simulink model "camber_control"  (R2025b)
settings: Solver=ode4  StartTime=0.0  StopTime=simin.Time.data(end)  FixedStep=0.01  RelTol=1e-3
model workspace (MAT data in the model file):
  simin.Car_CFL_q0.name = 'Car.CFL.q0'
  simin.Car_CFL_q0.unit = 'm'
  simin.Car_CFL_q0.nstates = 0
  simin.Car_CFL_q0.firststate = 0
  simin.Car_CFL_q0.data = [-0.000886241672561 -0.000917865429074 -0.000943370396271 -0.000939193181694 -0.000899850332644 -0.000822894508019 -0.000713430286851 -0.000581348023843 -0.000436899543274 -0.000289270334179 -0.000146343198139 -1.46837728607e-05 ... (6000 elements, 1x6000)]
  simin.Car_CFL_q2.name = 'Car.CFL.q2'
  simin.Car_CFL_q2.unit = 'm'
  simin.Car_CFL_q2.nstates = 0
  simin.Car_CFL_q2.firststate = 0
  simin.Car_CFL_q2.data = [0 1.19206197269e-05 4.64434779133e-05 5.49509059056e-05 2.16799271584e-05 -2.95135832857e-05 -7.40940522519e-05 -0.000103421145468 -0.000119076255942 -0.000124738915474 -0.000123357822304 -0.000117349867651 ... (6000 elements, 1x6000)]
  simin.Car_CFL_rx.name = 'Car.CFL.rx'
  simin.Car_CFL_rx.unit = 'rad'
  simin.Car_CFL_rx.nstates = 0
  simin.Car_CFL_rx.firststate = 0
  simin.Car_CFL_rx.data = [-0.00065072166035 -0.000697329873219 -0.000728137092665 -0.000743675802369 -0.000721060263459 -0.000660504738335 -0.000585128553212 -0.000514992512763 -0.000457198155345 -0.000411092391005 -0.000374412920792 -0.000345494656358 ... (6000 elements, 1x6000)]
  simin.Car_CFL_rx_kin.name = 'Car.CFL.rx_kin'
  simin.Car_CFL_rx_kin.unit = 'rad'
  simin.Car_CFL_rx_kin.nstates = 0
  simin.Car_CFL_rx_kin.firststate = 0
  simin.Car_CFL_rx_kin.data = [-0.000256283470662 -0.000262994930381 -0.000266255956376 -0.000264801376034 -0.000259094289504 -0.000244981871219 -0.000220309899305 -0.000186673511053 -0.000147291997564 -0.000105385945062 -6.36886106804e-05 -2.44687053055e-05 ... (6000 elements, 1x6000)]
  simin.Car_CFR_q0.name = 'Car.CFR.q0'
  simin.Car_CFR_q0.unit = 'm'
  simin.Car_CFR_q0.nstates = 0
  simin.Car_CFR_q0.firststate = 0
  simin.Car_CFR_q0.data = [-0.00088600104209 -0.000906234839931 -0.00091196334688 -0.000886910362169 -0.000833748606965 -0.000755003711674 -0.000651485286653 -0.00052521424368 -0.000380918907467 -0.000225870186114 -6.8379813456e-05 8.35821483633e-05 ... (6000 elements, 1x6000)]
  simin.Car_CFR_q2.name = 'Car.CFR.q2'
  simin.Car_CFR_q2.unit = 'm'
  simin.Car_CFR_q2.nstates = 0
  simin.Car_CFR_q2.firststate = 0
  simin.Car_CFR_q2.data = [0 1.19206197269e-05 4.64434779133e-05 5.49509059056e-05 2.16799271584e-05 -2.95135832857e-05 -7.40940522519e-05 -0.000103421145468 -0.000119076255942 -0.000124738915474 -0.000123357822304 -0.000117349867651 ... (6000 elements, 1x6000)]
  simin.Car_CFR_rx.name = 'Car.CFR.rx'
  simin.Car_CFR_rx.unit = 'rad'
  simin.Car_CFR_rx.nstates = 0
  simin.Car_CFR_rx.firststate = 0
  simin.Car_CFR_rx.data = [0.000650721834973 0.000686773331836 0.000667747866828 0.000635246396996 0.000626600987744 0.000641913560685 0.00065922603244 0.000660477147903 0.000641017919406 0.00060491275508 0.000558351166546 0.000506999145728 ... (6000 elements, 1x6000)]
  simin.Car_CFR_rx_kin.name = 'Car.CFR.rx_kin'
  simin.Car_CFR_rx_kin.unit = 'rad'
  simin.Car_CFR_rx_kin.nstates = 0
  simin.Car_CFR_rx_kin.firststate = 0
  simin.Car_CFR_rx_kin.data = [0.000256283325143 0.000263447727775 0.000270785414614 0.000265596871031 0.000246212730417 0.000216875007027 0.000181285664439 0.000141187847476 9.76538649411e-05 5.22338450537e-05 6.92095409249e-06 -3.62966420653e-05 ... (6000 elements, 1x6000)]
  simin.Car_CRL_q0.name = 'Car.CRL.q0'
  simin.Car_CRL_q0.unit = 'm'
  simin.Car_CRL_q0.nstates = 0
  simin.Car_CRL_q0.firststate = 0
  simin.Car_CRL_q0.data = [-0.000690113112796 -0.000714901543688 -0.00076236174209 -0.000825292314403 -0.000905930181034 -0.00100995623507 -0.00113963766489 -0.00129249203019 -0.00146282243077 -0.00164327386301 -0.00182610820048 -0.00200403272174 ... (6000 elements, 1x6000)]
  simin.Car_CRL_rx.name = 'Car.CRL.rx'
  simin.Car_CRL_rx.unit = 'rad'
  simin.Car_CRL_rx.nstates = 0
  simin.Car_CRL_rx.firststate = 0
  simin.Car_CRL_rx.data = [0.0257834587246 0.0257766991854 0.0257623307407 0.025743059814 0.0257183741778 0.0256865043193 0.0256465747952 0.0255992393941 0.0255462061614 0.0254897512496 0.0254323091358 0.0253761913627 ... (6000 elements, 1x6000)]
  simin.Car_CRL_rx_kin.name = 'Car.CRL.rx_kin'
  simin.Car_CRL_rx_kin.unit = 'rad'
  simin.Car_CRL_rx_kin.nstates = 0
  simin.Car_CRL_rx_kin.firststate = 0
  simin.Car_CRL_rx_kin.data = [0.0257834587246 0.0257766991854 0.0257623307407 0.025743059814 0.0257183741778 0.0256865043193 0.0256465747952 0.0255992393941 0.0255462061614 0.0254897512496 0.0254323091358 0.0253761913627 ... (6000 elements, 1x6000)]
  simin.Car_CRR_q0.name = 'Car.CRR.q0'
  simin.Car_CRR_q0.unit = 'm'
  simin.Car_CRR_q0.nstates = 0
  simin.Car_CRR_q0.firststate = 0
  simin.Car_CRR_q0.data = [-0.000689887441695 -0.000704726902768 -0.000737457768992 -0.000787679164205 -0.000858748855535 -0.000955924740992 -0.00108009413816 -0.0012272374006 -0.00139052153099 -0.0015617198078 -0.00173251959495 -0.00189547974151 ... (6000 elements, 1x6000)]
  simin.Car_CRR_rx.name = 'Car.CRR.rx'
  simin.Car_CRR_rx.unit = 'rad'
  simin.Car_CRR_rx.nstates = 0
  simin.Car_CRR_rx.firststate = 0
  simin.Car_CRR_rx.data = [-0.0257834605873 -0.0257794577628 -0.0257697012275 -0.0257545150816 -0.0257329326123 -0.0257032830268 -0.0256651025265 -0.0256195366383 -0.025568658486 -0.0255150310695 -0.0254612769932 -0.0254097674042 ... (6000 elements, 1x6000)]
  simin.Car_CRR_rx_kin.name = 'Car.CRR.rx_kin'
  simin.Car_CRR_rx_kin.unit = 'rad'
  simin.Car_CRR_rx_kin.nstates = 0
  simin.Car_CRR_rx_kin.firststate = 0
  simin.Car_CRR_rx_kin.data = [-0.0257834605873 -0.0257794577628 -0.0257697012275 -0.0257545150816 -0.0257329326123 -0.0257032830268 -0.0256651025265 -0.0256195366383 -0.025568658486 -0.0255150310695 -0.0254612769932 -0.0254097674042 ... (6000 elements, 1x6000)]
  simin.Car_CamberFL.name = 'Car.CamberFL'
  simin.Car_CamberFL.unit = 'rad'
  simin.Car_CamberFL.nstates = 0
  simin.Car_CamberFL.firststate = 0
  simin.Car_CamberFL.data = [0.00065072166035 0.000697329873219 0.000728137092665 0.000743675802369 0.000721060263459 0.000660504738335 0.000585128553212 0.000514992512763 0.000457198155345 0.000411092391005 0.000374412920792 0.000345494656358 ... (6000 elements, 1x6000)]
  simin.Car_CamberFR.name = 'Car.CamberFR'
  simin.Car_CamberFR.unit = 'rad'
  simin.Car_CamberFR.nstates = 0
  simin.Car_CamberFR.firststate = 0
  simin.Car_CamberFR.data = [0.000650721834973 0.000686773331836 0.000667747866828 0.000635246396996 0.000626600987744 0.000641913560685 0.00065922603244 0.000660477147903 0.000641017919406 0.00060491275508 0.000558351166546 0.000506999145728 ... (6000 elements, 1x6000)]
  simin.Car_CamberRL.name = 'Car.CamberRL'
  simin.Car_CamberRL.unit = 'rad'
  simin.Car_CamberRL.nstates = 0
  simin.Car_CamberRL.firststate = 0
  simin.Car_CamberRL.data = [-0.0257834587246 -0.0257766991854 -0.0257623307407 -0.025743059814 -0.0257183741778 -0.0256865043193 -0.0256465747952 -0.0255992393941 -0.0255462061614 -0.0254897512496 -0.0254323091358 -0.0253761913627 ... (6000 elements, 1x6000)]
  simin.Car_CamberRR.name = 'Car.CamberRR'
  simin.Car_CamberRR.unit = 'rad'
  simin.Car_CamberRR.nstates = 0
  simin.Car_CamberRR.firststate = 0
  simin.Car_CamberRR.data = [-0.0257834605873 -0.0257794577628 -0.0257697012275 -0.0257545150816 -0.0257329326123 -0.0257032830268 -0.0256651025265 -0.0256195366383 -0.025568658486 -0.0255150310695 -0.0254612769932 -0.0254097674042 ... (6000 elements, 1x6000)]
  simin.Car_DampFL_Frc.name = 'Car.DampFL.Frc'
  simin.Car_DampFL_Frc.unit = 'N'
  simin.Car_DampFL_Frc.nstates = 0
  simin.Car_DampFL_Frc.firststate = 0
  simin.Car_DampFL_Frc.data = [0 -9.93723297119 -4.40193367004 2.46527552605 8.21194553375 13.9642562866 18.4993839264 21.4081287384 22.7783069611 22.8000087738 21.6752319336 19.6104412079 ... (6000 elements, 1x6000)]
  simin.Car_DampFR_Frc.name = 'Car.DampFR.Frc'
  simin.Car_DampFR_Frc.unit = 'N'
  simin.Car_DampFR_Frc.nstates = 0
  simin.Car_DampFR_Frc.firststate = 0
  simin.Car_DampFR_Frc.data = [0 -5.6295466423 0.758005857468 5.51679039001 9.56676769257 13.4871988297 17.2829322815 20.6506958008 23.1178970337 24.3567123413 24.2942562103 23.0426483154 ... (6000 elements, 1x6000)]
  simin.Car_DampRL_Frc.name = 'Car.DampRL.Frc'
  simin.Car_DampRL_Frc.unit = 'N'
  simin.Car_DampRL_Frc.nstates = 0
  simin.Car_DampRL_Frc.firststate = 0
  simin.Car_DampRL_Frc.data = [0 -11.4901485443 -17.2899723053 -22.3062095642 -28.6704177856 -36.8323631287 -45.1161651611 -52.1466941833 -57.0556297302 -59.4691352844 -59.3767662048 -56.9993171692 ... (6000 elements, 1x6000)]
  simin.Car_DampRR_Frc.name = 'Car.DampRR.Frc'
  simin.Car_DampRR_Frc.unit = 'N'
  simin.Car_DampRR_Frc.nstates = 0
  simin.Car_DampRR_Frc.firststate = 0
  simin.Car_DampRR_Frc.data = [0 -7.11860799789 -12.5467271805 -18.5251407623 -25.9145946503 -34.8317947388 -43.3664627075 -50.1834983826 -54.5467147827 -56.1566467285 -55.1185531616 -51.7984848022 ... (6000 elements, 1x6000)]
  simin.Car_KinPitchCenter_L_x.name = 'Car.KinPitchCenter_L.x'
  simin.Car_KinPitchCenter_L_x.unit = 'm'
  simin.Car_KinPitchCenter_L_x.nstates = 0
  simin.Car_KinPitchCenter_L_x.firststate = 0
  simin.Car_KinPitchCenter_L_x.data = [0.504387140274 0.504145979881 0.502829492092 0.50243729353 0.503771483898 0.505480468273 0.506275355816 0.505792319775 0.504277765751 0.502096116543 0.499556958675 0.496920496225 ... (6000 elements, 1x6000)]
  simin.Car_KinPitchCenter_L_x_1.name = 'Car.KinPitchCenter_L.x_1'
  simin.Car_KinPitchCenter_L_x_1.unit = 'm'
  simin.Car_KinPitchCenter_L_x_1.nstates = 0
  simin.Car_KinPitchCenter_L_x_1.firststate = 0
  simin.Car_KinPitchCenter_L_x_1.data = [1.61338853836 1.59092903137 1.58962082863 1.58924043179 1.59058964252 1.59231734276 1.59313392639 1.59267413616 1.591183424 1.5890250206 1.58650791645 1.58389151096 ... (6000 elements, 1x6000)]
  simin.Car_KinPitchCenter_L_y_1.name = 'Car.KinPitchCenter_L.y_1'
  simin.Car_KinPitchCenter_L_y_1.unit = 'm'
  simin.Car_KinPitchCenter_L_y_1.nstates = 0
  simin.Car_KinPitchCenter_L_y_1.firststate = 0
  simin.Car_KinPitchCenter_L_y_1.data = [0.812810838223 0.812809169292 0.812811613083 0.812808275223 0.812796890736 0.812784671783 0.812776327133 0.812772095203 0.812770485878 0.812770247459 0.812770962715 0.812772035599 ... (6000 elements, 1x6000)]
  simin.Car_KinPitchCenter_L_z.name = 'Car.KinPitchCenter_L.z'
  simin.Car_KinPitchCenter_L_z.unit = 'm'
  simin.Car_KinPitchCenter_L_z.nstates = 0
  simin.Car_KinPitchCenter_L_z.firststate = 0
  simin.Car_KinPitchCenter_L_z.data = [0.203027188778 0.202923417091 0.202380791306 0.202208995819 0.202729135752 0.203393802047 0.203682735562 0.203450009227 0.202796339989 0.201870456338 0.200799122453 0.199689269066 ... (6000 elements, 1x6000)]
  simin.Car_KinPitchCenter_L_z_1.name = 'Car.KinPitchCenter_L.z_1'
  simin.Car_KinPitchCenter_L_z_1.unit = 'm'
  simin.Car_KinPitchCenter_L_z_1.nstates = 0
  simin.Car_KinPitchCenter_L_z_1.firststate = 0
  simin.Car_KinPitchCenter_L_z_1.data = [0.181995794177 0.181882992387 0.181306168437 0.181078404188 0.18152192235 0.182088240981 0.182257398963 0.181886732578 0.181082576513 0.18000048399 0.178774029016 0.177516147494 ... (6000 elements, 1x6000)]
  simin.Car_KinPitchCenter_R_x.name = 'Car.KinPitchCenter_R.x'
  simin.Car_KinPitchCenter_R_x.unit = 'm'
  simin.Car_KinPitchCenter_R_x.nstates = 0
  simin.Car_KinPitchCenter_R_x.firststate = 0
  simin.Car_KinPitchCenter_R_x.data = [0.504397392273 0.505248427391 0.507386863232 0.507622241974 0.505006432533 0.500874817371 0.496615886688 0.492787390947 0.489389508963 0.486331731081 0.483586013317 0.481158673763 ... (6000 elements, 1x6000)]
  simin.Car_KinPitchCenter_R_x_1.name = 'Car.KinPitchCenter_R.x_1'
  simin.Car_KinPitchCenter_R_x_1.unit = 'm'
  simin.Car_KinPitchCenter_R_x_1.nstates = 0
  simin.Car_KinPitchCenter_R_x_1.firststate = 0
  simin.Car_KinPitchCenter_R_x_1.data = [1.61339890957 1.59203147888 1.59417819977 1.59442532063 1.59182441235 1.58771181107 1.58347499371 1.57967054844 1.57629740238 1.57326376438 1.57054078579 1.56813430786 ... (6000 elements, 1x6000)]
  simin.Car_KinPitchCenter_R_y_1.name = 'Car.KinPitchCenter_R.y_1'
  simin.Car_KinPitchCenter_R_y_1.unit = 'm'
  simin.Car_KinPitchCenter_R_y_1.nstates = 0
  simin.Car_KinPitchCenter_R_y_1.firststate = 0
  simin.Car_KinPitchCenter_R_y_1.data = [-0.812810778618 -0.81280374527 -0.812789201736 -0.812784314156 -0.812790989876 -0.812801122665 -0.812808871269 -0.812813222408 -0.812815070152 -0.812815129757 -0.81281375885 -0.81281119585 ... (6000 elements, 1x6000)]
  simin.Car_KinPitchCenter_R_z.name = 'Car.KinPitchCenter_R.z'
  simin.Car_KinPitchCenter_R_z.unit = 'm'
  simin.Car_KinPitchCenter_R_z.nstates = 0
  simin.Car_KinPitchCenter_R_z.firststate = 0
  simin.Car_KinPitchCenter_R_z.data = [0.203031331301 0.203367009759 0.204212725163 0.204290360212 0.203219071031 0.201533898711 0.199791356921 0.198215171695 0.196806028485 0.195529073477 0.194375172257 0.193349123001 ... (6000 elements, 1x6000)]
  simin.Car_KinPitchCenter_R_z_1.name = 'Car.KinPitchCenter_R.z_1'
  simin.Car_KinPitchCenter_R_z_1.unit = 'm'
  simin.Car_KinPitchCenter_R_z_1.nstates = 0
  simin.Car_KinPitchCenter_R_z_1.firststate = 0
  simin.Car_KinPitchCenter_R_z_1.data = [0.181999951601 0.182334989309 0.183165609837 0.18320658803 0.1820730865 0.180297747254 0.178439259529 0.176727846265 0.175172701478 0.17374765873 0.172451332211 0.17129470408 ... (6000 elements, 1x6000)]
  simin.Car_KinRollCenter_F_x_1.name = 'Car.KinRollCenter_F.x_1'
  simin.Car_KinRollCenter_F_x_1.unit = 'm'
  simin.Car_KinRollCenter_F_x_1.nstates = 0
  simin.Car_KinRollCenter_F_x_1.firststate = 0
  simin.Car_KinRollCenter_F_x_1.data = [4.08391618729 4.06163883209 4.06161642075 4.06162166595 4.06163978577 4.06166744232 4.06170082092 4.06173610687 4.06177186966 4.06180620193 4.06183862686 4.0618686676 ... (6000 elements, 1x6000)]
  simin.Car_KinRollCenter_F_y.name = 'Car.KinRollCenter_F.y'
  simin.Car_KinRollCenter_F_y.unit = 'm'
  simin.Car_KinRollCenter_F_y.nstates = 0
  simin.Car_KinRollCenter_F_y.firststate = 0
  simin.Car_KinRollCenter_F_y.data = [2.19647540689e-06 0.000294854107779 0.00112901662942 0.0014056772925 0.000699118536431 -0.000498738780152 -0.00161035964265 -0.00237797247246 -0.00280151120387 -0.00295699504204 -0.0029179379344 -0.00274892663583 ... (6000 elements, 1x6000)]
  simin.Car_KinRollCenter_F_y_1.name = 'Car.KinRollCenter_F.y_1'
  simin.Car_KinRollCenter_F_y_1.unit = 'm'
  simin.Car_KinRollCenter_F_y_1.nstates = 0
  simin.Car_KinRollCenter_F_y_1.firststate = 0
  simin.Car_KinRollCenter_F_y_1.data = [2.197422873e-06 0.000292710261419 0.00111504783854 0.00137761724181 0.000672959838994 -0.000503810239024 -0.0015871420037 -0.002331224503 -0.00274047674611 -0.00289000780322 -0.00285091577098 -0.00268561020494 ... (6000 elements, 1x6000)]
  simin.Car_KinRollCenter_F_z.name = 'Car.KinRollCenter_F.z'
  simin.Car_KinRollCenter_F_z.unit = 'm'
  simin.Car_KinRollCenter_F_z.nstates = 0
  simin.Car_KinRollCenter_F_z.firststate = 0
  simin.Car_KinRollCenter_F_z.data = [0.106545142829 0.106592223048 0.106616981328 0.106594122946 0.106523387134 0.10640425235 0.106240332127 0.10604160279 0.105820596218 0.105590626597 0.105364337564 0.105152584612 ... (6000 elements, 1x6000)]
  simin.Car_KinRollCenter_F_z_1.name = 'Car.KinRollCenter_F.z_1'
  simin.Car_KinRollCenter_F_z_1.unit = 'm'
  simin.Car_KinRollCenter_F_z_1.nstates = 0
  simin.Car_KinRollCenter_F_z_1.firststate = 0
  simin.Car_KinRollCenter_F_z_1.data = [0.0853210985661 0.0853668823838 0.0853964090347 0.085396669805 0.0853713303804 0.0853234902024 0.0852591320872 0.0851852670312 0.0851074233651 0.085029900074 0.0849560722709 0.0848886221647 ... (6000 elements, 1x6000)]
  simin.Car_KinRollCenter_R_x_1.name = 'Car.KinRollCenter_R.x_1'
  simin.Car_KinRollCenter_R_x_1.unit = 'm'
  simin.Car_KinRollCenter_R_x_1.nstates = 0
  simin.Car_KinRollCenter_R_x_1.firststate = 0
  simin.Car_KinRollCenter_R_x_1.data = [1.10899782181 1.08677971363 1.086789608 1.08680522442 1.08682656288 1.08685445786 1.08688807487 1.08692574501 1.08696520329 1.08700454235 1.08704209328 1.08707654476 ... (6000 elements, 1x6000)]
  simin.Car_KinRollCenter_R_y.name = 'Car.KinRollCenter_R.y'
  simin.Car_KinRollCenter_R_y.unit = 'm'
  simin.Car_KinRollCenter_R_y.nstates = 0
  simin.Car_KinRollCenter_R_y.firststate = 0
  simin.Car_KinRollCenter_R_y.data = [-6.46729887421e-08 -3.79616576538e-05 -0.000128477113321 -0.000218971676077 -0.000285943562631 -0.000326405162923 -0.000350159883965 -0.000371785165044 -0.00040298118256 -0.000450946361525 -0.000519107619766 -0.000607466325164 ... (6000 elements, 1x6000)]
  simin.Car_KinRollCenter_R_y_1.name = 'Car.KinRollCenter_R.y_1'
  simin.Car_KinRollCenter_R_y_1.unit = 'm'
  simin.Car_KinRollCenter_R_y_1.nstates = 0
  simin.Car_KinRollCenter_R_y_1.firststate = 0
  simin.Car_KinRollCenter_R_y_1.data = [-6.4395990762e-08 -3.86120118492e-05 -0.000129369596834 -0.000219902343815 -0.00028688609018 -0.000327294197632 -0.000350904971128 -0.000372283160686 -0.000403118872782 -0.000450624676887 -0.000518255634233 -0.000606045883615 ... (6000 elements, 1x6000)]
  simin.Car_KinRollCenter_R_z.name = 'Car.KinRollCenter_R.z'
  simin.Car_KinRollCenter_R_z.unit = 'm'
  simin.Car_KinRollCenter_R_z.nstates = 0
  simin.Car_KinRollCenter_R_z.firststate = 0
  simin.Car_KinRollCenter_R_z.data = [0.0665587410331 0.0665603280067 0.0665664896369 0.0665797144175 0.0666007995605 0.0666303038597 0.0666679367423 0.0667121484876 0.066760532558 0.0668103843927 0.0668591335416 0.0669046789408 ... (6000 elements, 1x6000)]
  simin.Car_KinRollCenter_R_z_1.name = 'Car.KinRollCenter_R.z_1'
  simin.Car_KinRollCenter_R_z_1.unit = 'm'
  simin.Car_KinRollCenter_R_z_1.nstates = 0
  simin.Car_KinRollCenter_R_z_1.firststate = 0
  simin.Car_KinRollCenter_R_z_1.data = [0.0455666817725 0.0455627404153 0.0455382838845 0.0454909913242 0.045419190079 0.045320764184 0.0451966375113 0.0450519807637 0.0448944941163 0.0447327457368 0.0445747412741 0.0444271154702 ... (6000 elements, 1x6000)]
  simin.Car_Pitch.name = 'Car.Pitch'
  simin.Car_Pitch.unit = 'rad'
  simin.Car_Pitch.nstates = 0
  simin.Car_Pitch.firststate = 0
  simin.Car_Pitch.data = [-7.79904221417e-05 -7.52850028221e-05 -6.04344786552e-05 -2.87524653686e-05 2.16342832573e-05 9.28552399273e-05 0.000184569405974 0.000292906479444 0.000411794229876 0.000534347142093 0.000654049625155 0.000765463977586 ... (6000 elements, 1x6000)]
  simin.Car_PitchAcc.name = 'Car.PitchAcc'
  simin.Car_PitchAcc.unit = 'rad/s^2'
  simin.Car_PitchAcc.nstates = 0
  simin.Car_PitchAcc.firststate = 0
  simin.Car_PitchAcc.data = [-0.00852889381349 0.121664509177 0.168158859015 0.183013767004 0.209344476461 0.210217341781 0.173254683614 0.112931802869 0.0432517528534 -0.0232782959938 -0.0791946575046 -0.12137915194 ... (6000 elements, 1x6000)]
  simin.Car_PitchVel.name = 'Car.PitchVel'
  simin.Car_PitchVel.unit = 'rad/s'
  simin.Car_PitchVel.nstates = 0
  simin.Car_PitchVel.firststate = 0
  simin.Car_PitchVel.data = [-8.52889388625e-06 0.000697757815942 0.00219579669647 0.00398335745558 0.00594720616937 0.0080813486129 0.0100052338094 0.0114194946364 0.0121677154675 0.0122276162729 0.0116766653955 0.0106413085014 ... (6000 elements, 1x6000)]
  simin.Car_Roll.name = 'Car.Roll'
  simin.Car_Roll.unit = 'rad'
  simin.Car_Roll.nstates = 0
  simin.Car_Roll.firststate = 0
  simin.Car_Roll.data = [1.43921411677e-07 7.30765304979e-06 1.96193504962e-05 3.09518691211e-05 3.8966009015e-05 4.36614427599e-05 4.65610137326e-05 4.95717540616e-05 5.41080044059e-05 6.10112620052e-05 7.06324863131e-05 8.28800766612e-05 ... (6000 elements, 1x6000)]
  simin.Car_RollAcc.name = 'Car.RollAcc'
  simin.Car_RollAcc.unit = 'rad/s^2'
  simin.Car_RollAcc.nstates = 0
  simin.Car_RollAcc.firststate = 0
  simin.Car_RollAcc.data = [0.135388016701 0.0584235191345 -0.00935550685972 -0.0331188887358 -0.0355286933482 -0.020376265049 -0.000107629442937 0.0145972631872 0.0234513655305 0.0274394322187 0.0268719661981 0.0224712211639 ... (6000 elements, 1x6000)]
  simin.Car_RollVel.name = 'Car.RollVel'
  simin.Car_RollVel.unit = 'rad/s'
  simin.Car_RollVel.nstates = 0
  simin.Car_RollVel.firststate = 0
  simin.Car_RollVel.data = [0.00013538802159 0.00107662170194 0.00125746871345 0.000999151030555 0.000636012176983 0.00035703877802 0.000266080634901 0.000351245660568 0.000550257274881 0.000810600584373 0.00108493550215 0.00133225508034 ... (6000 elements, 1x6000)]
  simin.Car_SlipAngleFL.name = 'Car.SlipAngleFL'
  simin.Car_SlipAngleFL.unit = 'rad'
  simin.Car_SlipAngleFL.nstates = 0
  simin.Car_SlipAngleFL.firststate = 0
  simin.Car_SlipAngleFL.data = [0.00274525093846 0.00262049841695 0.0027533150278 0.00272545171902 0.00250543863513 0.00227329134941 0.00213159737177 0.00207538134418 0.00206845672801 0.00208716187626 0.00212029693648 0.00215951306745 ... (6000 elements, 1x6000)]
  simin.Car_SlipAngleFR.name = 'Car.SlipAngleFR'
  simin.Car_SlipAngleFR.unit = 'rad'
  simin.Car_SlipAngleFR.nstates = 0
  simin.Car_SlipAngleFR.firststate = 0
  simin.Car_SlipAngleFR.data = [-0.00274524791166 -0.00241396040656 -0.00218636821955 -0.0022307287436 -0.00249595101923 -0.00277927983552 -0.00295931030996 -0.00303354393691 -0.00303959334269 -0.00300525082275 -0.00294662476517 -0.00287613342516 ... (6000 elements, 1x6000)]
  simin.Car_SlipAngleRL.name = 'Car.SlipAngleRL'
  simin.Car_SlipAngleRL.unit = 'rad'
  simin.Car_SlipAngleRL.nstates = 0
  simin.Car_SlipAngleRL.firststate = 0
  simin.Car_SlipAngleRL.data = [0.0019979889039 0.00200495659374 0.00200151791796 0.00198903609999 0.00197318592109 0.00195616809651 0.00194171629846 0.00193085568026 0.00192299752962 0.00191747827921 0.00191350083333 0.00191024434753 ... (6000 elements, 1x6000)]
  simin.Car_SlipAngleRR.name = 'Car.SlipAngleRR'
  simin.Car_SlipAngleRR.unit = 'rad'
  simin.Car_SlipAngleRR.nstates = 0
  simin.Car_SlipAngleRR.firststate = 0
  simin.Car_SlipAngleRR.data = [-0.0019979889039 -0.00195998512208 -0.00194531306624 -0.00194091035519 -0.00193618691992 -0.00192808767315 -0.0019188785227 -0.00191189511679 -0.00191012339201 -0.00191501819063 -0.00192689360119 -0.00194531341549 ... (6000 elements, 1x6000)]
  simin.Car_SpringFL_Frc.name = 'Car.SpringFL.Frc'
  simin.Car_SpringFL_Frc.unit = 'N'
  simin.Car_SpringFL_Frc.nstates = 0
  simin.Car_SpringFL_Frc.firststate = 0
  simin.Car_SpringFL_Frc.data = [3699.37353516 3698.52294922 3697.69482422 3697.71899414 3698.77563477 3700.94433594 3704.09033203 3707.92749023 3712.15332031 3716.49487305 3720.71801758 3724.62646484 ... (6000 elements, 1x6000)]
  simin.Car_SpringFR_Frc.name = 'Car.SpringFR.Frc'
  simin.Car_SpringFR_Frc.unit = 'N'
  simin.Car_SpringFR_Frc.nstates = 0
  simin.Car_SpringFR_Frc.firststate = 0
  simin.Car_SpringFR_Frc.data = [3699.37548828 3698.82446289 3698.58496094 3699.23291016 3700.70776367 3702.93188477 3705.88891602 3709.52856445 3713.71972656 3718.25366211 3722.88623047 3727.38037109 ... (6000 elements, 1x6000)]
  simin.Car_SpringRL_Frc.name = 'Car.SpringRL.Frc'
  simin.Car_SpringRL_Frc.unit = 'N'
  simin.Car_SpringRL_Frc.nstates = 0
  simin.Car_SpringRL_Frc.firststate = 0
  simin.Car_SpringRL_Frc.data = [3300.99462891 3300.13378906 3298.30322266 3295.84838867 3292.70361328 3288.64379883 3283.55737305 3277.52734375 3270.77148438 3263.57983398 3256.26245117 3249.11352539 ... (6000 elements, 1x6000)]
  simin.Car_SpringRR_Frc.name = 'Car.SpringRR.Frc'
  simin.Car_SpringRR_Frc.unit = 'N'
  simin.Car_SpringRR_Frc.nstates = 0
  simin.Car_SpringRR_Frc.firststate = 0
  simin.Car_SpringRR_Frc.data = [3300.99658203 3300.48681641 3299.24389648 3297.30957031 3294.55981445 3290.78295898 3285.91943359 3280.11450195 3273.63354492 3266.80200195 3259.95410156 3253.39257812 ... (6000 elements, 1x6000)]
  simin.Car_StabiFL_Frc.name = 'Car.StabiFL.Frc'
  simin.Car_StabiFL_Frc.unit = 'N'
  simin.Car_StabiFL_Frc.nstates = 0
  simin.Car_StabiFL_Frc.firststate = 0
  simin.Car_StabiFL_Frc.data = [7.82602728577e-06 0.138030618429 0.413827478886 0.694055497646 0.865083992481 0.867504477501 0.764490902424 0.664155781269 0.642086148262 0.72485023737 0.906963646412 1.16916048527 ... (6000 elements, 1x6000)]
  simin.Car_StabiFR_Frc.name = 'Car.StabiFR.Frc'
  simin.Car_StabiFR_Frc.unit = 'N'
  simin.Car_StabiFR_Frc.nstates = 0
  simin.Car_StabiFR_Frc.firststate = 0
  simin.Car_StabiFR_Frc.data = [-7.82602728577e-06 -0.138030618429 -0.413827478886 -0.694055497646 -0.865083992481 -0.867504477501 -0.764490902424 -0.664155781269 -0.642086148262 -0.72485023737 -0.906963646412 -1.16916048527 ... (6000 elements, 1x6000)]
  simin.Car_StabiRL_Frc.name = 'Car.StabiRL.Frc'
  simin.Car_StabiRL_Frc.unit = 'N'
  simin.Car_StabiRL_Frc.nstates = 0
  simin.Car_StabiRL_Frc.firststate = 0
  simin.Car_StabiRL_Frc.data = [9.64909268077e-05 0.131720602512 0.35206502676 0.547254264355 0.695473074913 0.801495492458 0.885083138943 0.969595432281 1.0726429224 1.20764803886 1.38378286362 1.60394978523 ... (6000 elements, 1x6000)]
  simin.Car_StabiRR_Frc.name = 'Car.StabiRR.Frc'
  simin.Car_StabiRR_Frc.unit = 'N'
  simin.Car_StabiRR_Frc.nstates = 0
  simin.Car_StabiRR_Frc.firststate = 0
  simin.Car_StabiRR_Frc.data = [-9.64909268077e-05 -0.131720602512 -0.35206502676 -0.547254264355 -0.695473074913 -0.801495492458 -0.885083138943 -0.969595432281 -1.0726429224 -1.20764803886 -1.38378286362 -1.60394978523 ... (6000 elements, 1x6000)]
  simin.Car_SteerAngleFL.name = 'Car.SteerAngleFL'
  simin.Car_SteerAngleFL.unit = 'rad'
  simin.Car_SteerAngleFL.nstates = 0
  simin.Car_SteerAngleFL.firststate = 0
  simin.Car_SteerAngleFL.data = [-0.00274520018138 -0.00261072162539 -0.00273614027537 -0.00272827874869 -0.00252113584429 -0.00227158749476 -0.0020858021453 -0.00197293353267 -0.0019090451533 -0.00187749683391 -0.00187091040425 -0.00188293971587 ... (6000 elements, 1x6000)]
  simin.Car_SteerAngleFR.name = 'Car.SteerAngleFR'
  simin.Car_SteerAngleFR.unit = 'rad'
  simin.Car_SteerAngleFR.nstates = 0
  simin.Car_SteerAngleFR.firststate = 0
  simin.Car_SteerAngleFR.data = [0.00274519715458 0.00245770136826 0.00221033743583 0.00219813152216 0.00241411244497 0.00267922622152 0.00287288380787 0.00298104900867 0.00303049129434 0.003042408498 0.00302849058062 0.0029978682287 ... (6000 elements, 1x6000)]
  simin.Car_SteerAngleRL.name = 'Car.SteerAngleRL'
  simin.Car_SteerAngleRL.unit = 'rad'
  simin.Car_SteerAngleRL.nstates = 0
  simin.Car_SteerAngleRL.firststate = 0
  simin.Car_SteerAngleRL.data = [-0.00200000009499 -0.00200000009499 -0.00200000009499 -0.00200000009499 -0.00200000009499 -0.00200000009499 -0.00200000009499 -0.00200000009499 -0.00200000009499 -0.00200000009499 -0.00200000009499 -0.00200000009499 ... (6000 elements, 1x6000)]
  simin.Car_SteerAngleRR.name = 'Car.SteerAngleRR'
  simin.Car_SteerAngleRR.unit = 'rad'
  simin.Car_SteerAngleRR.nstates = 0
  simin.Car_SteerAngleRR.firststate = 0
  simin.Car_SteerAngleRR.data = [0.00200000009499 0.00200000009499 0.00200000009499 0.00200000009499 0.00200000009499 0.00200000009499 0.00200000009499 0.00200000009499 0.00200000009499 0.00200000009499 0.00200000009499 0.00200000009499 ... (6000 elements, 1x6000)]
  simin.Car_ax.name = 'Car.ax'
  simin.Car_ax.unit = 'm/s^2'
  simin.Car_ax.nstates = 0
  simin.Car_ax.firststate = 0
  simin.Car_ax.data = [-0.457714706659 -0.534652173519 -0.662542879581 -0.741676449776 -0.843408048153 -0.914272546768 -0.900144159794 -0.82865524292 -0.726453304291 -0.619308292866 -0.523603081703 -0.446811616421 ... (6000 elements, 1x6000)]
  simin.Car_ay.name = 'Car.ay'
  simin.Car_ay.unit = 'm/s^2'
  simin.Car_ay.nstates = 0
  simin.Car_ay.firststate = 0
  simin.Car_ay.data = [0.0283882785589 -0.0120470412076 -0.0242476686835 -0.0307025741786 -0.0163070317358 0.0105119002983 0.0332782119513 0.0458651073277 0.0503795333207 0.0500719510019 0.0471589565277 0.0429927967489 ... (6000 elements, 1x6000)]
  simin.Car_az.name = 'Car.az'
  simin.Car_az.unit = 'm/s^2'
  simin.Car_az.nstates = 0
  simin.Car_az.firststate = 0
  simin.Car_az.data = [1.57921946049 0.0678593143821 0.0510049164295 0.0390680357814 0.0383200794458 0.0183836277574 0.000795689527877 -0.0124301603064 -0.020629376173 -0.0241743065417 -0.0244926121086 -0.0227019377053 ... (6000 elements, 1x6000)]
  simin.Car_tx.name = 'Car.tx'
  simin.Car_tx.unit = 'm'
  simin.Car_tx.nstates = 0
  simin.Car_tx.firststate = 0
  simin.Car_tx.data = [2.61795282364 2.84016108513 3.0623190403 3.28441166878 3.50642991066 3.72836446762 3.9502081871 4.1719622612 4.39363288879 4.61523103714 4.83676624298 5.05824899673 ... (6000 elements, 1x6000)]
  simin.Car_ty.name = 'Car.ty'
  simin.Car_ty.unit = 'm'
  simin.Car_ty.nstates = 0
  simin.Car_ty.firststate = 0
  simin.Car_ty.data = [-5.5 -5.50000047684 -5.50000143051 -5.50000524521 -5.50001192093 -5.50001955032 -5.50002574921 -5.50002813339 -5.50002622604 -5.50001955032 -5.50000762939 -5.49999141693 ... (6000 elements, 1x6000)]
  simin.Car_tz.name = 'Car.tz'
  simin.Car_tz.unit = 'm'
  simin.Car_tz.nstates = 0
  simin.Car_tz.firststate = 0
  simin.Car_tz.data = [0.625109732151 0.62511330843 0.625121891499 0.625134706497 0.625151395798 0.62517118454 0.625193357468 0.625216901302 0.625240981579 0.625264883041 0.625288069248 0.625310182571 ... (6000 elements, 1x6000)]
  simin.Car_v.name = 'Car.v'
  simin.Car_v.unit = 'm/s'
  simin.Car_v.nstates = 0
  simin.Car_v.firststate = 0
  simin.Car_v.data = [22.2222213745 22.2189311981 22.2130565643 22.2060241699 22.1982498169 22.1894168854 22.1802577972 22.1715068817 22.1636238098 22.1568069458 22.1510219574 22.1461219788 ... (6000 elements, 1x6000)]
  simin.Steer_L_q.name = 'Steer.L.q'
  simin.Steer_L_q.unit = 'm'
  simin.Steer_L_q.nstates = 0
  simin.Steer_L_q.firststate = 0
  simin.Steer_L_q.data = [0 1.19206197269e-05 4.64434779133e-05 5.49509059056e-05 2.16799271584e-05 -2.95135832857e-05 -7.40940522519e-05 -0.000103421145468 -0.000119076255942 -0.000124738915474 -0.000123357822304 -0.000117349867651 ... (6000 elements, 1x6000)]
  simin.Steer_R_q.name = 'Steer.R.q'
  simin.Steer_R_q.unit = 'm'
  simin.Steer_R_q.nstates = 0
  simin.Steer_R_q.firststate = 0
  simin.Steer_R_q.data = [0 1.19206197269e-05 4.64434779133e-05 5.49509059056e-05 2.16799271584e-05 -2.95135832857e-05 -7.40940522519e-05 -0.000103421145468 -0.000119076255942 -0.000124738915474 -0.000123357822304 -0.000117349867651 ... (6000 elements, 1x6000)]
  simin.Steer_RL_q.name = 'Steer.RL.q'
  simin.Steer_RL_q.unit = 'm'
  simin.Steer_RL_q.nstates = 0
  simin.Steer_RL_q.firststate = 0
  simin.Steer_RL_q.data = [0 0 0 0 0 0 0 0 0 0 0 0 ... (6000 elements, 1x6000)]
  simin.Steer_RR_q.name = 'Steer.RR.q'
  simin.Steer_RR_q.unit = 'm'
  simin.Steer_RR_q.nstates = 0
  simin.Steer_RR_q.firststate = 0
  simin.Steer_RR_q.data = [0 0 0 0 0 0 0 0 0 0 0 0 ... (6000 elements, 1x6000)]
  simin.Time.name = 'Time'
  simin.Time.unit = 's'
  simin.Time.nstates = 0
  simin.Time.firststate = 0
  simin.Time.data = [0 0.01 0.02 0.03 0.04 0.05 0.06 0.07 0.08 0.09 0.1 0.11 ... (6000 elements, 1x6000)]
undefined symbols (not defined in the file): camberMapFL, compression, compression_FL, compression_FR, distance_to_pitch_center_front, steer, steering_rack_displacement_FL, steering_rack_displacement_FR, track_width_front, track_width_rear, wheelbase
settings Model: DataDictionary=vehicleData.sldd  EnableAccessToBaseWorkspace=off  Creator=marce  LastModifiedBy=marcelkaminski

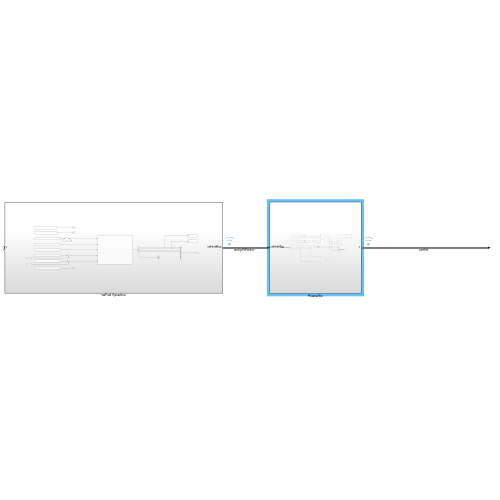
[thumbnail: Simulink's stored preview of the top-level diagram]
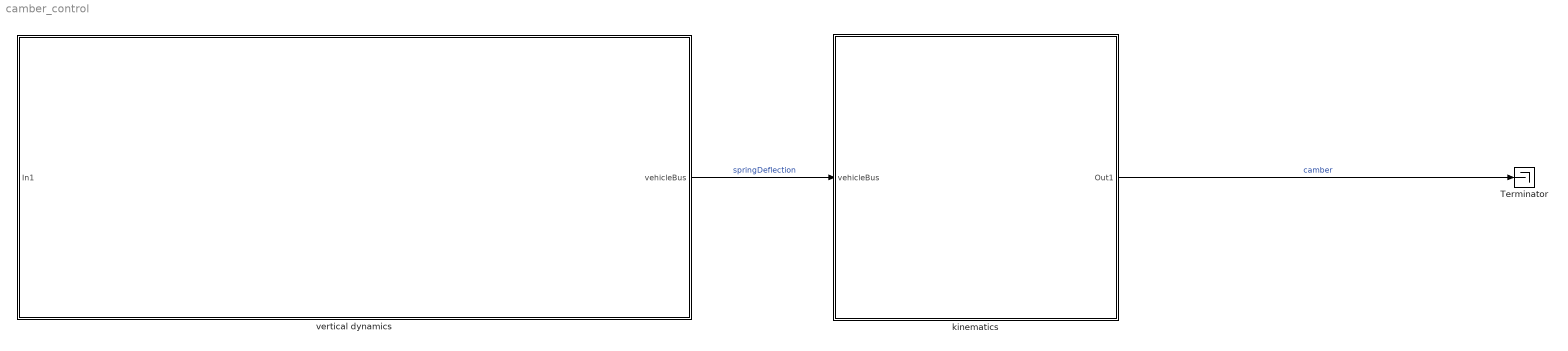
== system camber_control ==
  Terminator : Terminator
  kinematics : Subsystem
  vertical dynamics : Subsystem
  wires:
  vertical dynamics/1(vehicleBus) -> kinematics/1(vehicleBus)  "springDeflection"
  kinematics/1(Out1) -> Terminator/1  "camber"

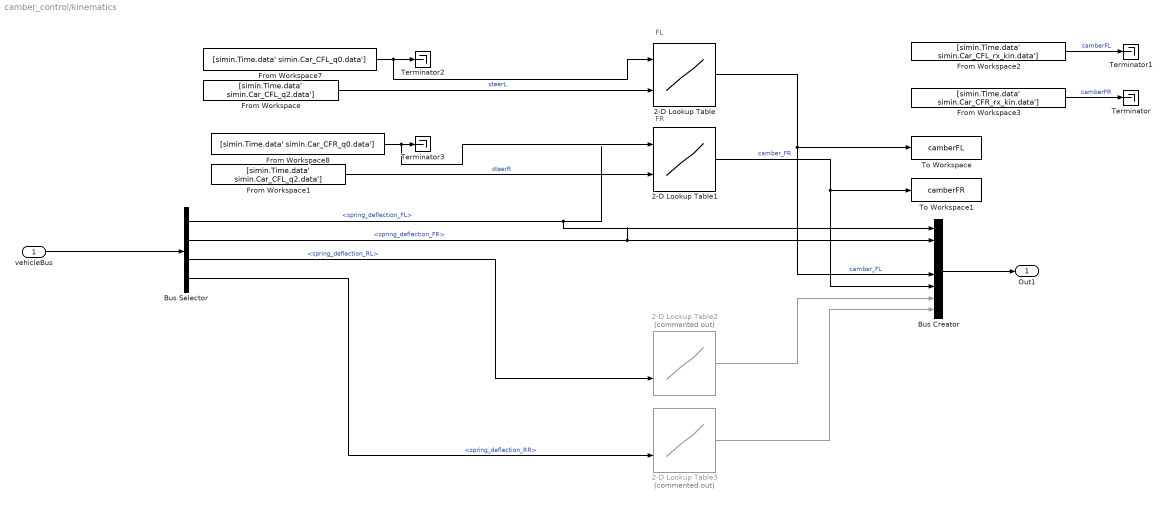
== system camber_control/kinematics ==
  note: FL
  note: FR
  vehicleBus : Inport  OutDataTypeStr=Bus: camberControlBus
  2-D Lookup Table : Lookup_n-D  BreakpointsForDimension1=compression_FL  BreakpointsForDimension2=steering_rack_displacement_FL  Table=camber_map_FL'  InterpMethod=Linear Lagrange  InternalRulePriority=Speed  RndMeth=Simplest
      settings: InputPortMap=u0,u1
  2-D Lookup Table1 : Lookup_n-D  BreakpointsForDimension1=compression_FR  BreakpointsForDimension2=steering_rack_displacement_FR  Table=camber_map_FR'  InterpMethod=Linear Lagrange  InternalRulePriority=Speed  RndMeth=Simplest
      settings: InputPortMap=u0,u1
  2-D Lookup Table2 : Lookup_n-D  Commented=on  BreakpointsForDimension1=steer.*10^3'  BreakpointsForDimension2=compression.*10^3  Table=camberMapFL  InternalRulePriority=Speed  RndMeth=Simplest
      settings: InputPortMap=u0,u1
  2-D Lookup Table3 : Lookup_n-D  Commented=on  BreakpointsForDimension1=steer.*10^3'  BreakpointsForDimension2=compression.*10^3  Table=camberMapFL  InternalRulePriority=Speed  RndMeth=Simplest
      settings: InputPortMap=u0,u1
  Bus Creator : BusCreator  Inputs=8  OutDataTypeStr=Bus: camberControlBus
      settings: InheritFromInputs=off
  Bus Selector : BusSelector  OutputSignals=spring_deflection_FL,spring_deflection_FR,spring_deflection_RL,spring_deflection_RR
  From Workspace : FromWorkspace  VariableName=[simin.Time.data' simin.Car_CFL_q2.data']
  From Workspace1 : FromWorkspace  VariableName=[simin.Time.data' simin.Car_CFL_q2.data']
  From Workspace2 : FromWorkspace  VariableName=[simin.Time.data' simin.Car_CFL_rx_kin.data']
  From Workspace3 : FromWorkspace  VariableName=[simin.Time.data' simin.Car_CFR_rx_kin.data']
  From Workspace7 : FromWorkspace  VariableName=[simin.Time.data' simin.Car_CFL_q0.data']
  From Workspace8 : FromWorkspace  VariableName=[simin.Time.data' simin.Car_CFR_q0.data']
  Terminator{,1..3} (4 alike) : Terminator
  To Workspace : ToWorkspace  VariableName=camberFL  SampleTime=0.01
      settings: Save2DSignal=2-D array (concatenate along first dimension)
  To Workspace1 : ToWorkspace  VariableName=camberFR  SampleTime=0.01
      settings: Save2DSignal=2-D array (concatenate along first dimension)
  Out1 : Outport  OutDataTypeStr=Bus: camberControlBus
  wires:
  2-D Lookup Table/1 -> Bus Creator/5, To Workspace/1  "camber_FL"
  2-D Lookup Table1/1 -> Bus Creator/6, To Workspace1/1  "camber_FR"
  vehicleBus/1 -> Bus Selector/1
  Bus Selector/1 -> Bus Creator/1  "<spring_deflection_FL>"
  Bus Selector/2 -> Bus Creator/2  "<spring_deflection_FR>"
  Bus Selector/3 -> 2-D Lookup Table2/2  "<spring_deflection_RL>"
  Bus Selector/4 -> 2-D Lookup Table3/2  "<spring_deflection_RR>"
  Bus Creator/1 -> Out1/1
  2-D Lookup Table2/1 -> Bus Creator/7
  2-D Lookup Table3/1 -> Bus Creator/8
  From Workspace/1 -> 2-D Lookup Table/2  "steerL"
  From Workspace7/1 -> 2-D Lookup Table/1, Terminator2/1
  From Workspace3/1 -> Terminator/1  "camberFR"
  From Workspace2/1 -> Terminator1/1  "camberFL"
  From Workspace8/1 -> 2-D Lookup Table1/1, Terminator3/1
  From Workspace1/1 -> 2-D Lookup Table1/2  "steerR"

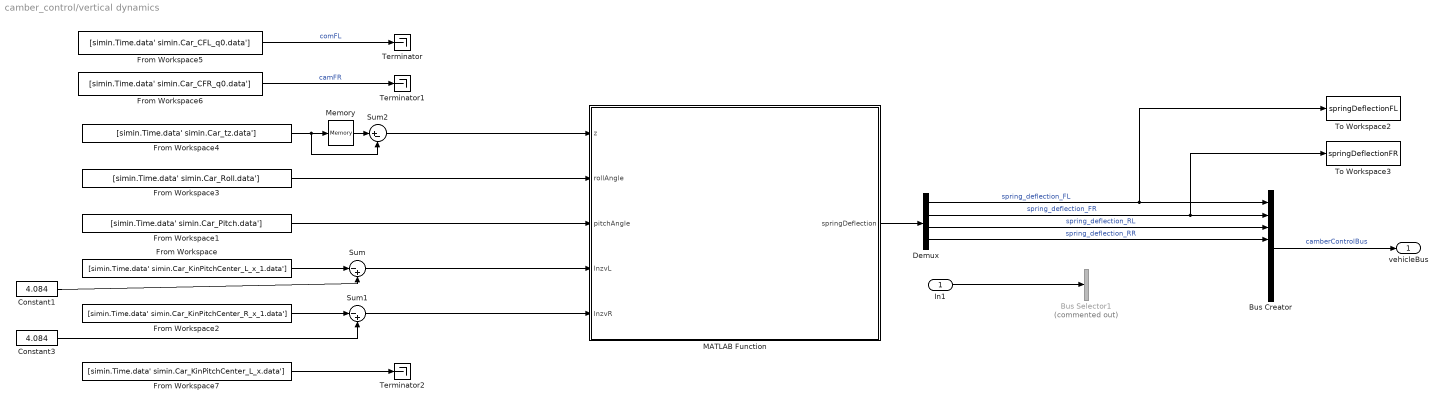
== system camber_control/vertical dynamics ==
  In1 : Inport  OutDataTypeStr=Bus: camberControlBus
  Bus Creator : BusCreator  Inputs=8  OutDataTypeStr=Bus: camberControlBus
  Bus Selector1 : BusSelector  Commented=on  OutputSignals=signal1,signal2
  Constant1 : Constant  Value=4.084
  Constant3 : Constant  Value=4.084
  Demux : Demux
  From Workspace : FromWorkspace  VariableName=[simin.Time.data' simin.Car_KinPitchCenter_L_x_1.data']
  From Workspace1 : FromWorkspace  VariableName=[simin.Time.data' simin.Car_Pitch.data']
  From Workspace2 : FromWorkspace  VariableName=[simin.Time.data' simin.Car_KinPitchCenter_R_x_1.data']
  From Workspace3 : FromWorkspace  VariableName=[simin.Time.data' simin.Car_Roll.data']
  From Workspace4 : FromWorkspace  VariableName=[simin.Time.data' simin.Car_tz.data']
  From Workspace5 : FromWorkspace  VariableName=[simin.Time.data' simin.Car_CFL_q0.data']
  From Workspace6 : FromWorkspace  VariableName=[simin.Time.data' simin.Car_CFR_q0.data']
  From Workspace7 : FromWorkspace  VariableName=[simin.Time.data' simin.Car_KinPitchCenter_L_x.data']
  MATLAB Function : MATLAB Function  TreatAsAtomicUnit=on
  Memory : Memory  InitialCondition=simin.Car_tz.data(1)'
  Sum : Sum  Inputs=|-+
  Sum1 : Sum  Inputs=|-+
  Sum2 : Sum  Inputs=|+-
  Terminator : Terminator
  Terminator1 : Terminator
  Terminator2 : Terminator
  To Workspace2 : ToWorkspace  VariableName=springDeflectionFL  SampleTime=0.01
      settings: Save2DSignal=2-D array (concatenate along first dimension)
  To Workspace3 : ToWorkspace  VariableName=springDeflectionFR  SampleTime=0.01
      settings: Save2DSignal=2-D array (concatenate along first dimension)
  vehicleBus : Outport  OutDataTypeStr=double
  wires:
  MATLAB Function/1(springDeflection) -> Demux/1
  Demux/1 -> To Workspace2/1, Bus Creator/1  "spring_deflection_FL"
  Demux/2 -> To Workspace3/1, Bus Creator/2  "spring_deflection_FR"
  Bus Creator/1 -> vehicleBus/1  "camberControlBus"
  Demux/3 -> Bus Creator/3  "spring_deflection_RL"
  Demux/4 -> Bus Creator/4  "spring_deflection_RR"
  In1/1 -> Bus Selector1/1
  From Workspace/1 -> Sum/1
  Constant1/1 -> Sum/2
  From Workspace2/1 -> Sum1/1
  Constant3/1 -> Sum1/2
  From Workspace4/1 -> Memory/1, Sum2/2
  From Workspace5/1 -> Terminator/1  "comFL"
  Sum2/1 -> MATLAB Function/1(z)
  From Workspace6/1 -> Terminator1/1  "camFR"
  Sum/1 -> MATLAB Function/4(lnzvL)
  Memory/1 -> Sum2/1
  Sum1/1 -> MATLAB Function/5(lnzvR)
  From Workspace7/1 -> Terminator2/1
  From Workspace1/1 -> MATLAB Function/3(pitchAngle)
  From Workspace3/1 -> MATLAB Function/2(rollAngle)

== matlab function camber_control/vertical dynamics/MATLAB Function ==
  data: z input double; rollAngle input; springDeflection output; pitchAngle input; wheelbase parameter; distance_to_pitch_center_front parameter; track_width_rear parameter; track_width_front parameter; lnzvL input; lnzvR input
function springDeflection = wheel_elevation(z, rollAngle, pitchAngle, ...
    wheelbase, distance_to_pitch_center_front, track_width_rear, track_width_front, lnzvL, lnzvR)

l = wheelbase;
sv = track_width_front;
sh = track_width_rear;
%lnzv = distance_to_pitch_center_front;

z1 = z - sin(rollAngle) * (sv/2) + sin(pitchAngle) * lnzvL;     % vorne links
z2 = z + sin(rollAngle) * (sv/2) + sin(pitchAngle) * lnzvR;     % vorne rechts
z3 = z - sin(rollAngle) * (sh/2) - sin(pitchAngle) * (l-lnzvL); % hinten links
z4 = z + sin(rollAngle) * (sh/2) - sin(pitchAngle) * (l-lnzvR); % hinten rechts

springDeflection = [z1, z2, z3, z4];
